simulink model "model_podstawowy_2015a"  (R2015a)
settings: Solver=ode45  SolverMode=SingleTasking  StartTime=0.0  StopTime=15  RelTol=1e-3
undefined symbols (not defined in the file): g, J, K_reg, L, m, M, Q2, x_konc, x_pocz
settings Model: CovMetricSettings=dwe  CovHtmlReporting=off  covSaveCumulativeToWorkspaceVar=off  CovSaveSingleToWorkspaceVar=off  CovExternalEMLEnable=on  Creator=maelstro  LastModifiedBy=maelstro
settings DataIOCC: LimitDataPoints=off  SaveFormat=Dataset  ReturnWorkspaceOutputs=on
settings DebuggingCC: SFUnexpectedBacktrackingDiag=error  SFNoUnconditionalDefaultTransitionDiag=error
settings HardwareCC: ProdBitPerPointer=64  ProdLargestAtomicFloat=Float  ProdIntDivRoundTo=Zero  ProdEndianess=LittleEndian  ProdHWDeviceType=Specified
settings ModelReferenceCC: PropagateSignalLabelsOutOfModel=on
settings SFSimCC: SimUseLocalCustomCode=on
settings RTWCC: RTWUseLocalCustomCode=on
settings GRTTargetCC: TargetLangStandard=C99 (ISO)

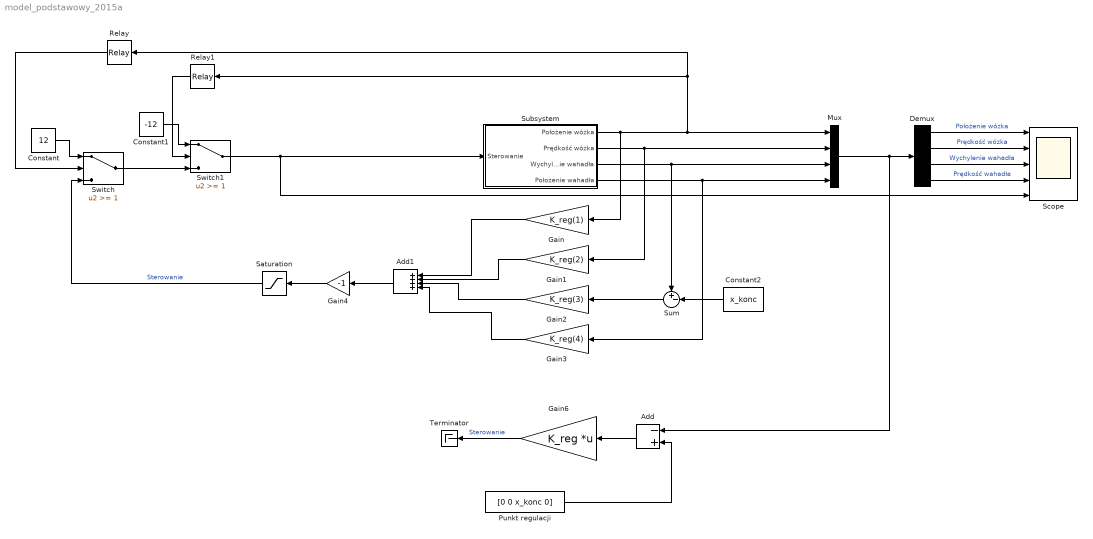
== system model_podstawowy_2015a ==
  Add : Sum  Inputs=-+
  Add1 : Sum  Inputs=++++
  Constant : Constant  Value=12
  Constant1 : Constant  Value=-12
  Constant2 : Constant  Value=x_konc
  Demux : Demux
  Gain : Gain  Gain=K_reg(1)
  Gain1 : Gain  Gain=K_reg(2)
  Gain2 : Gain  Gain=K_reg(3)
  Gain3 : Gain  Gain=K_reg(4)
  Gain4 : Gain  Gain=-1
  Gain6 : Gain  Gain=K_reg  Multiplication=Matrix(K*u) (u vector)
  Mux : Mux
  Punkt regulacji : Constant  Value=[0 0 x_konc 0]  VectorParams1D=off
  Relay : Relay  OnSwitchValue=0.7  OffSwitchValue=0.6
  Relay1 : Relay  OnSwitchValue=-0.6  OffSwitchValue=-0.7  OnOutputValue=0  OffOutputValue=1
  Saturation : Saturate  UpperLimit=12  LowerLimit=-12
  Scope : Scope  NumInputPorts=5
      settings: TimeRange=auto  MaxDataPoints=5000  SaveToWorkspace=off  SaveName=ScopeData  YMin=-0.05807~-0.33449~2.90915~-3.10992~-5  YMax=0.5226~0.83444~3.23361~13.67888~5  SampleTime=-1
  Subsystem : Subsystem
  Sum : Sum  Inputs=+-|
  Switch : Switch  Threshold=1
  Switch1 : Switch  Threshold=1
  Terminator : Terminator
  wires:
  Mux/1 -> Add/1, Demux/1
  Punkt regulacji/1 -> Add/2
  Subsystem/2(Prędkość wózka) -> Gain1/1, Mux/2
  Subsystem/3(Wychylenie wahadła) -> Sum/1, Mux/3
  Subsystem/4(Położenie wahadła) -> Gain3/1, Mux/4
  Demux/1 -> Scope/1  "Położenie wózka"
  Demux/2 -> Scope/2  "Prędkość wózka"
  Demux/3 -> Scope/3  "Wychylenie wahadła"
  Demux/4 -> Scope/4  "Prędkość wahadła"
  Gain6/1 -> Terminator/1  "Sterowanie"
  Add/1 -> Gain6/1
  Relay/1 -> Switch/2
  Constant/1 -> Switch/1
  Subsystem/1(Położenie wózka) -> Gain/1, Relay/1, Relay1/1, Mux/1
  Relay1/1 -> Switch1/2
  Constant1/1 -> Switch1/1
  Switch/1 -> Switch1/3
  Saturation/1 -> Switch/3  "Sterowanie"
  Switch1/1 -> Scope/5, Subsystem/1(Sterowanie)
  Gain/1 -> Add1/1
  Gain1/1 -> Add1/2
  Gain2/1 -> Add1/3
  Gain3/1 -> Add1/4
  Sum/1 -> Gain2/1
  Constant2/1 -> Sum/2
  Add1/1 -> Gain4/1
  Gain4/1 -> Saturation/1

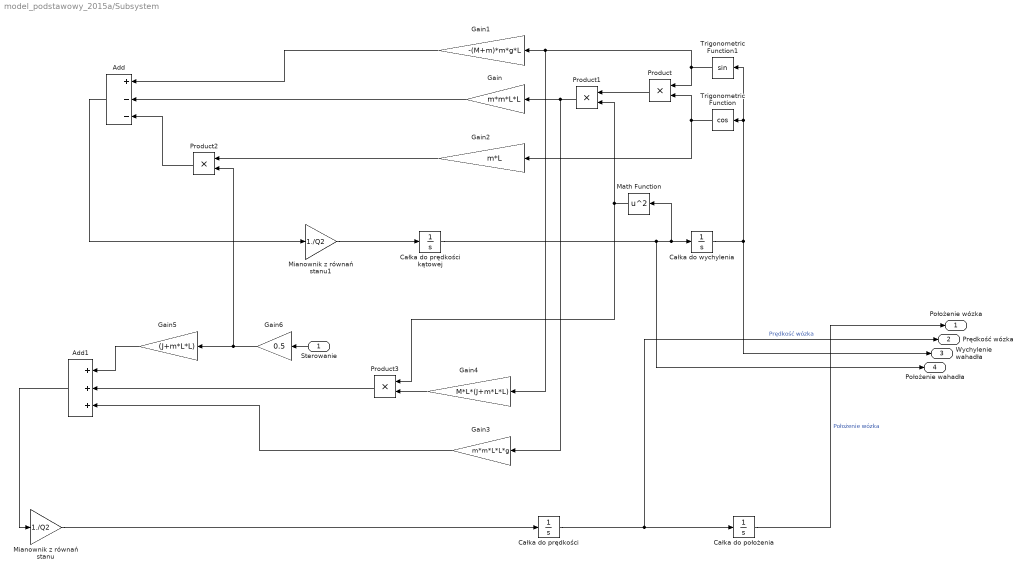
== system model_podstawowy_2015a/Subsystem ==
  Sterowanie : Inport
  Add : Sum  Inputs=+--
  Add1 : Sum  Inputs=+++
  Całka do położenia : Integrator
  Całka do prędkości : Integrator
  Całka do prędkości kątowej : Integrator
  Całka do wychylenia : Integrator  InitialCondition=x_pocz
  Gain : Gain  Gain=m*m*L*L
  Gain1 : Gain  Gain=-(M+m)*m*g*L
  Gain2 : Gain  Gain=m*L
  Gain3 : Gain  Gain=m*m*L*L*g
  Gain4 : Gain  Gain=M*L*(J+m*L*L)
  Gain5 : Gain  Gain=(J+m*L*L)
  Gain6 : Gain  Gain=0.5
  Math Function : Math  Operator=square  SaturateOnIntegerOverflow=on
  Mianownik z równań stanu : Gain  Gain=1./Q2
  Mianownik z równań stanu1 : Gain  Gain=1./Q2
  Product{,1..3} (4 alike) : Product
  Trigonometric Function : Trigonometry  Operator=cos
  Trigonometric Function1 : Trigonometry
  Położenie wózka : Outport
  Prędkość wózka : Outport  Port=2
  Wychylenie wahadła : Outport  Port=3
  Położenie wahadła : Outport  Port=4
  wires:
  Add1/1 -> Mianownik z równań stanu/1
  Add/1 -> Mianownik z równań stanu1/1
  Całka do prędkości/1 -> Prędkość wózka/1, Całka do położenia/1  "Prędkość wózka"
  Math Function/1 -> Product1/2, Product3/1
  Gain4/1 -> Product3/2
  Sterowanie/1 -> Gain6/1
  Product3/1 -> Add1/2
  Trigonometric Function/1 -> Gain2/1, Product/2
  Gain2/1 -> Product2/1
  Product1/1 -> Gain/1, Gain3/1
  Całka do wychylenia/1 -> Wychylenie wahadła/1, Trigonometric Function1/1, Trigonometric Function/1
  Całka do położenia/1 -> Położenie wózka/1  "Położenie wózka"
  Mianownik z równań stanu/1 -> Całka do prędkości/1
  Trigonometric Function1/1 -> Product/1, Gain4/1, Gain1/1
  Mianownik z równań stanu1/1 -> Całka do prędkości kątowej/1
  Gain/1 -> Add/2
  Gain1/1 -> Add/1
  Product/1 -> Product1/1
  Product2/1 -> Add/3
  Gain3/1 -> Add1/3
  Całka do prędkości kątowej/1 -> Położenie wahadła/1, Math Function/1, Całka do wychylenia/1
  Gain5/1 -> Add1/1
  Gain6/1 -> Product2/2, Gain5/1
